simulink model "testing_C_functions_doubles_substituting_every_function"  (R2020b)
settings: Solver=FixedStepAuto  StartTime=0.0  StopTime=10  FixedStep=Ts  RelTol=1e-3
undefined symbols (not defined in the file or in its folder): A_frq_step, A_phase_step, DiscIntNeverNeededParam, f_rad, k_phi, ki, kp, N, t_frq_step, t_phase_step, Ts, V_g, var_noise
libraries: bach_library x24, simulink x16, dspsrcs4 x1
(part 1 of 2)
settings Model: Creator=Kasper Laustsen  LastModifiedBy=Kasper Laustsen
settings SFSimCC: SimCustomHeaderCode=|
  | #include "PLL_doubled.h"
  | #include "MAF_doubled.h"
settings SFSimCC: SimUserSources=|
  | PLL_doubled.c
  | MAF_doubled.c

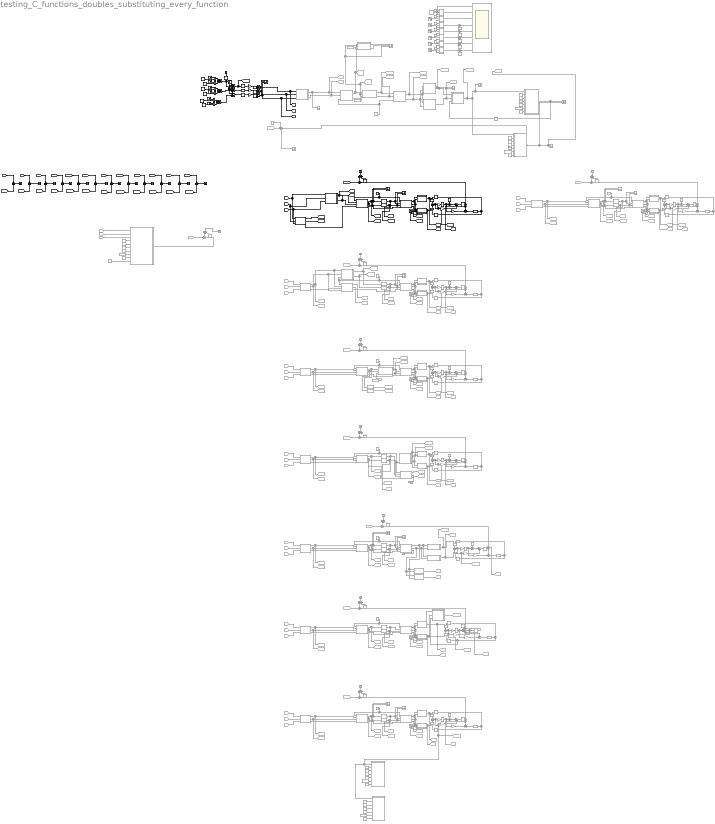
== system testing_C_functions_doubles_substituting_every_function ==
  note: Testing abc_to_alpha_beta
  note: TESTING abc_to_alphabeta
  note: MAF seems to be the limiting factor in terms of the code.
      | Experiment with changing the code inside of it to enable full simulation
  note: Noise
  note: Phase-jump
  note: Input signal incl. noise and phase- and frequency jump
  note: Frequency-jump
  note: MAF seems to be the limiting factor in terms of the code.
      | Experiment with changing the code inside of it to enable full simulation
  note: theta_pll
  note: theta_grid
  note: theta_pll
  note: theta_grid
  note: TESTING alphabeta_to_dq
  note: theta_pll
  note: theta_grid
  note: theta_grid
  note: theta_pll
  note: TESTING MAF
  note: theta_grid
  note: theta_pll
  note: TESTING dq_to_alphabeta
  note: theta_grid
  note: theta_pll
  note: TESTING cos_grid and sin_grid
  note: theta_grid
  note: theta_pll
  note: TESTING phase_detector
  note: theta_grid
  note: theta_pll
  note: TESTING pi_controller
  note: theta_grid
  note: theta_pll
  note: TRUE SIMULATION MODEL WITH DELAY
  Add{,1..5,7..10} (10 alike) : Sum
  Add{6,11..17} (8 alike) : Sum  Commented=on
  Chirp4 : dspsrcs4/Chirp  Commented=on  sweep=Linear  mode=Bidirectional  f0=0  f1=100  t1=2  Tsweep=2  phase=0  Ts=Ts  spf=1  datatype=Single  OutputFrames=off
  Constant{1..2,24,26,34,36,38,40,42,44,46,48} (12 alike) : Constant  Commented=on  Value=f_rad
  Constant{6,10,25,47,52} (5 alike) : Constant  Commented=on  Value=Ts
  Constant11 : Constant  Commented=on  Value=pi/2
  Constant12 : Constant  Commented=on  Value=6
  Constant13 : Constant  Commented=on  Value=10
  Constant14 : Constant  Commented=on  Value=8
  Constant{15..18,21..23} (7 alike) : Constant  Commented=on  Value=200
  Constant19 : Constant  Commented=on  Value=2
  Constant20 : Constant  Commented=on  Value=4
  Constant27 : Constant  Value=f_rad
  Constant28 : Constant  Value=-pi/2
  Constant{3,7,29,49,53} (5 alike) : Constant  Commented=on  Value=ki
  Constant{4,8,30,50,54} (5 alike) : Constant  Commented=on  Value=kp
  Constant{5,9,31,51,55} (5 alike) : Constant  Commented=on  Value=k_phi
  Constant{32..33,35,37,39,41,43,45} (8 alike) : Constant  Commented=on  Value=-pi/2
  Cos1 : Trigonometry  Operator=cos
  Cos{2..8} (7 alike) : Trigonometry  Commented=on  Operator=cos
  Delay : Delay  Commented=on  DelayLength=1  SampleTime=Ts
  Delay{1,3..8} (7 alike) : Delay  Commented=on  DelayLength=1
  Delay2 : Delay  DelayLength=1
  Derivative : Derivative
  Digital Clock{1..15} (15 alike) : DigitalClock  Commented=on  SampleTime=Ts
  Discrete FIR Filter{1,3,5..16} (14 alike) : DiscreteFir  Commented=on  Coefficients=[ones(1,round(N)).*1/N]  SampleTime=Ts
  Discrete FIR Filter2 : DiscreteFir  Coefficients=[ones(1,round(N)).*1/N]  SampleTime=Ts
  Discrete FIR Filter4 : DiscreteFir  Coefficients=[ones(1,round(N)).*1/N]  SampleTime=Ts
  Discrete-Time Integrator{1..2,5..16} (14 alike) : DiscreteIntegrator  Commented=on  IntegratorMethod=Integration: Trapezoidal  SampleTime=-1  ICPrevOutput=DiscIntNeverNeededParam  ICPrevScaledInput=DiscIntNeverNeededParam
  Discrete-Time Integrator3 : DiscreteIntegrator  IntegratorMethod=Integration: Trapezoidal  SampleTime=-1  ICPrevOutput=DiscIntNeverNeededParam  ICPrevScaledInput=DiscIntNeverNeededParam
  Discrete-Time Integrator4 : DiscreteIntegrator  IntegratorMethod=Integration: Trapezoidal  SampleTime=-1  ICPrevOutput=DiscIntNeverNeededParam  ICPrevScaledInput=DiscIntNeverNeededParam
  From{6,10,37,41,45,49,53,57} (8 alike) : From  Commented=on  GotoTag=B
  From{7,11,38,42,46,50,54,58} (8 alike) : From  Commented=on  GotoTag=C
  From{3,8,36,39,43,47,51,55,59} (9 alike) : From  Commented=on  GotoTag=phA_angle
  From{5,9,40,44,48,52,56,60} (8 alike) : From  Commented=on
  Gain{10..11,14,17,20,23,26} (7 alike) : Gain  Commented=on  Gain=k_phi
  Gain{2,12,15,18,21,24,27} (7 alike) : Gain  Commented=on  Gain=kp
  Gain{6,13,16,19,22,25,28} (7 alike) : Gain  Commented=on  Gain=ki
  Gain3 : Gain  Gain=V_g
  Gain4 : Gain  Gain=V_g
  Gain5 : Gain  Gain=V_g
  Gain7 : Gain  Gain=kp
  Gain8 : Gain  Gain=ki
  Gain9 : Gain  Gain=k_phi
  Goto{10,55,68,81,94,114} (6 alike) : Goto  Commented=on  GotoTag=d_pre_MAF
  Goto{40,48,61,87,100,107} (6 alike) : Goto  Commented=on  GotoTag=beta2
  Goto{41,49,62,75,88,101,108} (7 alike) : Goto  Commented=on  GotoTag=cosGrid
  Goto{5,50,63,76,89,102,109} (7 alike) : Goto  Commented=on  GotoTag=alpha1
  Goto{6,51,64,77,90,103,110} (7 alike) : Goto  Commented=on  GotoTag=sinGrid
  Goto{7,52,65,78,91,104,111} (7 alike) : Goto  Commented=on  GotoTag=anglePll
  Goto{8,53,66,79,92,105,112} (7 alike) : Goto  Commented=on  GotoTag=phaseError
  Goto{9,54,67,80,93,106,113} (7 alike) : Goto  Commented=on  GotoTag=beta1
  Goto{11,56,69,82,95,115} (6 alike) : Goto  Commented=on  GotoTag=q_pre_MAF
  Goto{12,44,57,70,83,96,116} (7 alike) : Goto  Commented=on  GotoTag=d_post_MAF
  Goto{38,45,58,71,84,97,117} (7 alike) : Goto  Commented=on  GotoTag=q_post_MAF
  Goto{39,46,59,85,98,118} (6 alike) : Goto  Commented=on  GotoTag=alpha2
  Goto13 : Goto  Commented=on  GotoTag=alpha1_C
  Goto14 : Goto  Commented=on  GotoTag=sinGrid_C
  Goto15 : Goto  Commented=on  GotoTag=anglePll_C
  Goto16 : Goto  Commented=on  GotoTag=phaseError_C
  Goto17 : Goto  Commented=on  GotoTag=beta1_C
  Goto18 : Goto  Commented=on  GotoTag=d_pre_MAF_C
  Goto19 : Goto  Commented=on  GotoTag=q_pre_MAF_C
  Goto20 : Goto  Commented=on  GotoTag=d_post_MAF_C
  Goto21 : Goto  Commented=on  GotoTag=q_post_MAF_C
  Goto22 : Goto  Commented=on  GotoTag=alpha2_C
  Goto23 : Goto  Commented=on  GotoTag=beta2_C
  Goto24 : Goto  Commented=on  GotoTag=cosGrid_C
  Goto42 : Goto  Commented=on  GotoTag=d_post_MAF_C
  Goto43 : Goto  Commented=on  GotoTag=q_post_MAF_C
  Goto47 : Goto  Commented=on  GotoTag=d_pre_MAF_C
  Goto60 : Goto  Commented=on  GotoTag=q_pre_MAF_C
  Goto72 : Goto  Commented=on  GotoTag=sinGrid_C
  Goto73 : Goto  Commented=on  GotoTag=alpha2_C
  Goto74 : Goto  Commented=on  GotoTag=cosGrid_C
  Goto86 : Goto  Commented=on  GotoTag=beta2_C
  Goto99 : Goto  Commented=on  GotoTag=phaseError_C
  MATLAB Function1 : MATLAB Function  Commented=on  TreatAsAtomicUnit=on
  MATLAB Function10 : MATLAB Function  Commented=on  TreatAsAtomicUnit=on
  MATLAB Function11 : MATLAB Function  Commented=on  TreatAsAtomicUnit=on
  MATLAB Function12 : MATLAB Function  Commented=on  TreatAsAtomicUnit=on
  MATLAB Function13 : MATLAB Function  Commented=on  TreatAsAtomicUnit=on
  MATLAB Function14 : MATLAB Function  Commented=on  TreatAsAtomicUnit=on
  MATLAB Function15 : MATLAB Function  Commented=on  TreatAsAtomicUnit=on
  MATLAB Function16 : MATLAB Function  Commented=on  TreatAsAtomicUnit=on
  MATLAB Function17 : MATLAB Function  Commented=on  TreatAsAtomicUnit=on
  MATLAB Function18 : MATLAB Function  Commented=on  TreatAsAtomicUnit=on
  MATLAB Function19 : MATLAB Function  TreatAsAtomicUnit=on
  MATLAB Function2 : MATLAB Function  Commented=on  TreatAsAtomicUnit=on
  MATLAB Function20 : MATLAB Function  TreatAsAtomicUnit=on
  MATLAB Function21 : MATLAB Function  Commented=on  TreatAsAtomicUnit=on
  MATLAB Function22 : MATLAB Function  Commented=on  TreatAsAtomicUnit=on
  MATLAB Function23 : MATLAB Function  Commented=on  TreatAsAtomicUnit=on
  MATLAB Function24 : MATLAB Function  Commented=on  TreatAsAtomicUnit=on
  MATLAB Function25 : MATLAB Function  Commented=on  TreatAsAtomicUnit=on
  MATLAB Function26 : MATLAB Function  Commented=on  TreatAsAtomicUnit=on
  MATLAB Function27 : MATLAB Function  Commented=on  TreatAsAtomicUnit=on
  MATLAB Function28 : MATLAB Function  Commented=on  TreatAsAtomicUnit=on
  MATLAB Function29 : MATLAB Function  Commented=on  TreatAsAtomicUnit=on
  MATLAB Function3 : MATLAB Function  Commented=on  TreatAsAtomicUnit=on
  MATLAB Function30 : MATLAB Function  Commented=on  TreatAsAtomicUnit=on
  MATLAB Function31 : MATLAB Function  Commented=on  TreatAsAtomicUnit=on
  MATLAB Function32 : MATLAB Function  Commented=on  TreatAsAtomicUnit=on
  MATLAB Function33 : MATLAB Function  Commented=on  TreatAsAtomicUnit=on
  MATLAB Function34 : MATLAB Function  Commented=on  TreatAsAtomicUnit=on
  MATLAB Function35 : MATLAB Function  Commented=on  TreatAsAtomicUnit=on
  MATLAB Function36 : MATLAB Function  Commented=on  TreatAsAtomicUnit=on
  MATLAB Function37 : MATLAB Function  Commented=on  TreatAsAtomicUnit=on
  MATLAB Function38 : MATLAB Function  Commented=on  TreatAsAtomicUnit=on
  MATLAB Function39 : MATLAB Function  Commented=on  TreatAsAtomicUnit=on
  MATLAB Function4 : MATLAB Function  Commented=on  TreatAsAtomicUnit=on
  MATLAB Function40 : MATLAB Function  Commented=on  TreatAsAtomicUnit=on
  MATLAB Function41 : MATLAB Function  Commented=on  TreatAsAtomicUnit=on
  MATLAB Function42 : MATLAB Function  Commented=on  TreatAsAtomicUnit=on
  MATLAB Function43 : MATLAB Function  Commented=on  TreatAsAtomicUnit=on
  MATLAB Function5 : MATLAB Function  Commented=on  TreatAsAtomicUnit=on
  MATLAB Function6 : MATLAB Function  Commented=on  TreatAsAtomicUnit=on
  MATLAB Function7 : MATLAB Function  Commented=on  TreatAsAtomicUnit=on
  MATLAB Function8 : MATLAB Function  Commented=on  TreatAsAtomicUnit=on
  MATLAB Function9 : MATLAB Function  TreatAsAtomicUnit=on
  Matrix Multiply{1,10..22} (14 alike) : Product  Commented=on
  Matrix Multiply{2..9} (8 alike) : Product
  Random Number : RandomNumber  Variance=var_noise  SampleTime=Ts
  Random Number1 : RandomNumber  Variance=var_noise  Seed=1  SampleTime=Ts
  Random Number2 : RandomNumber  Variance=var_noise  Seed=2  SampleTime=Ts
  Scope : Scope  Commented=on  NumInputPorts=3
  Scope1 : Scope  Commented=on
  Scope2 : Scope  Commented=on  NumInputPorts=8
  Scope3 : Scope  Commented=on
  Scope4 : Scope  Commented=on
  Scope5 : Scope  Commented=on  NumInputPorts=2
  Scope6 : Scope  Commented=on  NumInputPorts=2
  Scope8 : Scope  Commented=on  NumInputPorts=2
  Sin{1,3..5} (4 alike) : Trigonometry
  Sin{2,6..11} (7 alike) : Trigonometry  Commented=on
  Sine Wave14 : Sin  Commented=on  Frequency=f_rad*2.6  Phase=pi/2  SampleTime=Ts
  Sine Wave15 : Sin  Commented=on  Frequency=f_rad*2.8  Phase=pi/2  SampleTime=Ts
  Sine Wave16 : Sin  Commented=on  Frequency=f_rad*3  Phase=pi/2  SampleTime=Ts
  Sine Wave22 : Sin  Commented=on  Frequency=f_rad*2  Phase=pi/2  SampleTime=Ts
  Sine Wave23 : Sin  Commented=on  Frequency=f_rad*2.2  Phase=pi/2  SampleTime=Ts
  Sine Wave24 : Sin  Commented=on  Frequency=f_rad*2.4  Phase=pi/2  SampleTime=Ts
  Step : Step  Time=t_frq_step  Before=1  After=0  SampleTime=0
  Step1 : Step  Time=t_frq_step  SampleTime=0
  Step2 : Step  Time=t_frq_step  Before=1  After=0  SampleTime=0
  Step3 : Step  Time=t_frq_step  SampleTime=0
  Step4 : Step  Time=t_frq_step  Before=1  After=0  SampleTime=0
  Step5 : Step  Time=t_frq_step  SampleTime=0
  Sum : Sum  Commented=on  Inputs=+-|-
  Sum{1..4,9,15,33,38,43,48,53,58} (12 alike) : Sum  Commented=on  Inputs=|++
  Sum{10..14,16..22,25} (13 alike) : Sum  Inputs=+|-
  Sum23 : Sum  Inputs=-|+
  Sum24 : Sum  Inputs=++|
  Sum26 : Sum  Inputs=|++
  Sum27 : Sum  Inputs=+-|
  Sum{28..29,34,39,44,49,54} (7 alike) : Sum  Commented=on  Inputs=+-|
  Sum{6,30,35,40,45,50,55} (7 alike) : Sum  Commented=on  Inputs=-|+
  Sum{7,31,36,41,46,51,56} (7 alike) : Sum  Commented=on  Inputs=++|
  Sum{5,8,32,37,42,47,52,57} (8 alike) : Sum  Commented=on  Inputs=+|-
  Terminator{,2..15} (15 alike) : Terminator
  Terminator{1,16..29} (15 alike) : Terminator  Commented=on
  a_frq : simulink/Sources/Ramp  slope=f_rad  start=0  InitialOutput=0
  a_frq_step : simulink/Sources/Ramp  slope=f_rad*A_frq_step  start=t_frq_step  InitialOutput=t_frq_step*f_rad
  abc_to_alphabeta1 : bach_library/abc_to_alphabeta  SystemSampleTime=-1  VariantActivationTime=update diagram  Latency=0  AutoFrameSizeCalculation=off
  abc_to_alphabeta{2..8} (7 alike) : bach_library/abc_to_alphabeta  Commented=on  SystemSampleTime=-1  VariantActivationTime=update diagram  Latency=0  AutoFrameSizeCalculation=off
  alphabeta_to_dq1 : bach_library/alphabeta_to_dq  SystemSampleTime=-1  VariantActivationTime=update diagram  Latency=0  AutoFrameSizeCalculation=off
  alphabeta_to_dq{2..8} (7 alike) : bach_library/alphabeta_to_dq  Commented=on  SystemSampleTime=-1  VariantActivationTime=update diagram  Latency=0  AutoFrameSizeCalculation=off
  b_frq : simulink/Sources/Ramp  slope=f_rad  start=0  InitialOutput=-pi*2/3
  b_frq_step : simulink/Sources/Ramp  slope=f_rad*A_frq_step  start=t_frq_step  InitialOutput=t_frq_step*f_rad-pi*2/3
  c_frq : simulink/Sources/Ramp  slope=f_rad  start=0  InitialOutput=pi*2/3
  c_frq_step : simulink/Sources/Ramp  slope=f_rad*A_frq_step  start=t_frq_step  InitialOutput=t_frq_step*f_rad+pi*2/3
  dq_to_alphabeta1 : bach_library/dq_to_alphabeta  SystemSampleTime=-1  VariantActivationTime=update diagram  Latency=0  AutoFrameSizeCalculation=off
  dq_to_alphabeta{2..8} (7 alike) : bach_library/dq_to_alphabeta  Commented=on  SystemSampleTime=-1  VariantActivationTime=update diagram  Latency=0  AutoFrameSizeCalculation=off
  nominal frq{,1,3..9} (9 alike) : simulink/Sources/Ramp  Commented=on  slope=f_rad  start=0  InitialOutput=0
  nominal frq2 : simulink/Sources/Ramp  slope=f_rad  start=0  InitialOutput=0
  phase-jump : Step  Time=t_phase_step  After=A_phase_step  SampleTime=0
  phases : Scope  NumInputPorts=3
  post MAF1 : Scope  NumInputPorts=2
  post MAF{2,5,7..8} (4 alike) : Scope  Commented=on  NumInputPorts=2
  pre MAF1 : Scope  NumInputPorts=3
  pre MAF5 : Scope  Commented=on  NumInputPorts=3
  pre MAF7 : Scope  Commented=on  NumInputPorts=3
  pre MAF8 : Scope  Commented=on  NumInputPorts=3
  wires:
  MATLAB Function2/1(alpha) -> Goto13/1, MATLAB Function3/1(alpha), Scope4/1  "alpha1_C"
  Matrix Multiply4/1 -> Add5/2
  Matrix Multiply6/1 -> Add3/1
  Step2/1 -> Matrix Multiply2/1
  Matrix Multiply7/1 -> Add5/1
  Step4/1 -> Matrix Multiply4/1
  a_frq_step/1 -> Matrix Multiply6/2
  a_frq/1 -> Matrix Multiply5/2
  Step/1 -> Matrix Multiply5/1
  Sin5/1 -> Gain5/1  "theta_g"
  Gain5/1 -> Add9/1  "pc"
  Step5/1 -> Matrix Multiply7/1
  Matrix Multiply2/1 -> Add4/2
  Add5/1 -> Add2/2  "c_phase"
  c_frq_step/1 -> Matrix Multiply7/2
  b_frq/1 -> Matrix Multiply2/2
  Gain4/1 -> Add8/1  "pb"
  phase-jump/1 -> Add/1, Add2/1, Add1/1
  Add4/1 -> Add1/2  "b_phase"
  Add3/1 -> Add/2, Derivative/1  "a_phase"
  Random Number2/1 -> Add9/2
  b_frq_step/1 -> Matrix Multiply3/2
  Gain3/1 -> Add7/1  "pa"
  Sin4/1 -> Gain4/1  "theta_g"
  Add1/1 -> Sin4/1
  Random Number/1 -> Add7/2
  c_frq/1 -> Matrix Multiply4/2
  Add2/1 -> Sin5/1
  Random Number1/1 -> Add8/2
  Sin3/1 -> Gain3/1  "theta_g"
  Matrix Multiply5/1 -> Add3/2
  Step3/1 -> Matrix Multiply3/1
  Matrix Multiply3/1 -> Add4/1
  Step1/1 -> Matrix Multiply6/1
  Derivative/1 -> Terminator3/1  "omega_g"
  MATLAB Function4/2(beta) -> Goto23/1, MATLAB Function5/2(beta), MATLAB Function6/2(beta)  "beta2_C"
  MATLAB Function4/1(alpha) -> Goto22/1, MATLAB Function5/1(alpha), MATLAB Function6/1(alpha)  "alpha2_C"
  MATLAB Function5/1(cosGrid) -> Goto24/1, Scope8/1, MATLAB Function10/1(cosGrid)  "cosGrid_C"
  MATLAB Function6/1(sinGrid) -> MATLAB Function10/2(sinGrid), Scope8/2, Goto14/1  "sinGric_C"
  Constant2/1 -> MATLAB Function8/2(feedForward)
  Constant1/1 -> MATLAB Function7/2(feedForward)
  Digital Clock1/1 -> MATLAB Function7/6(t)
  Constant9/1 -> MATLAB Function8/5(kPhi)
  Digital Clock2/1 -> MATLAB Function8/6(t)
  Constant8/1 -> MATLAB Function8/4(kp)
  Constant6/1 -> MATLAB Function7/7(Ts)
  Constant7/1 -> MATLAB Function8/3(ki)
  Constant5/1 -> MATLAB Function7/5(kPhi)
  Constant10/1 -> MATLAB Function8/7(Ts)
  Constant4/1 -> MATLAB Function7/4(kp)
  Constant3/1 -> MATLAB Function7/3(ki)
  MATLAB Function7/1(anglePll) -> Sum/3, Scope6/2, Goto15/1, Scope5/1  "anglePll"
  nominal frq/1 -> MATLAB Function3/3(angle), MATLAB Function4/3(angle)
  MATLAB Function10/1(phaseError) -> Goto16/1, MATLAB Function7/1(phaseError), Scope3/1, MATLAB Function8/1(phaseError)  "phaseError_C"
  MATLAB Function8/1(anglePllComp) -> Delay/1, Scope6/1
  Constant11/1 -> Sum/2
  Sum/1 -> Scope1/1  "Angle_error_offset"
  MATLAB Function3/2(q) -> MATLAB Function18/2(sample2), Scope/3, MATLAB Function1/2(sample2), Goto19/1  "q_pre_MAF_C"
  Sum15/1 -> Scope2/8  "sin 150 Hz MAFed"
  Constant20/1 -> Sum2/2
  MATLAB Function12/1(y) -> Scope2/3  "sin 100 Hz MAFed"
  Constant19/1 -> Sum1/2
  MATLAB Function15/1(y) -> Sum3/1
  MATLAB Function14/1(y) -> Sum2/1
  Sine Wave14/1 -> MATLAB Function15/2(sample)
  Constant13/1 -> Sum15/2
  MATLAB Function17/1(y) -> Sum15/1
  MATLAB Function11/1(y) -> Scope2/2  "chirp MAFed"
  Sum2/1 -> Scope2/5  "sin 120 Hz MAFed"
  Sum3/1 -> Scope2/6  "sin 130 Hz MAFed"
  Chirp4/1 -> MATLAB Function11/2(sample), Scope2/1  "pa"
  Sine Wave22/1 -> MATLAB Function12/2(sample)
  Sine Wave15/1 -> MATLAB Function16/2(sample)
  MATLAB Function16/1(y) -> Sum4/1
  Sine Wave23/1 -> MATLAB Function13/2(sample)
  Constant14/1 -> Sum4/2
  Sum1/1 -> Scope2/4  "sin 110 Hz MAFed"
  MATLAB Function13/1(y) -> Sum1/1
  Sine Wave16/1 -> MATLAB Function17/2(sample)  "theta_g"
  Constant12/1 -> Sum3/2
  Sine Wave24/1 -> MATLAB Function14/2(sample)
  Sum4/1 -> Scope2/7  "sin 140 Hz MAFed"
  Constant15/1 -> MATLAB Function11/1(len)
  Digital Clock3/1 -> MATLAB Function11/3(t)
  Digital Clock4/1 -> MATLAB Function12/3(t)
  Constant16/1 -> MATLAB Function12/1(len)
  Digital Clock5/1 -> MATLAB Function13/3(t)
  Constant17/1 -> MATLAB Function13/1(len)
  Digital Clock6/1 -> MATLAB Function14/3(t)
  Constant18/1 -> MATLAB Function14/1(len)
  Digital Clock7/1 -> MATLAB Function15/3(t)
  Constant21/1 -> MATLAB Function15/1(len)
  Digital Clock8/1 -> MATLAB Function16/3(t)
  Constant22/1 -> MATLAB Function16/1(len)
  Digital Clock9/1 -> MATLAB Function17/3(t)
  Constant23/1 -> MATLAB Function17/1(len)
  MATLAB Function3/1(d) -> MATLAB Function18/1(sample1), Goto18/1, MATLAB Function1/1(sample1)  "d_pre_MAF_C"
  MATLAB Function18/1(y1) -> Goto20/1, MATLAB Function4/1(d)  "d_post_MAF_C"
  MATLAB Function18/2(y2) -> Goto21/1, MATLAB Function4/2(q)  "q_post_MAF_C"
  MATLAB Function2/2(beta) -> MATLAB Function3/2(beta), Goto17/1  "beta1_C"
  [alpha1] -> Sum10/1
  [alpha1_C] -> Sum10/2
  [beta1] -> Sum11/1
  [beta1_C] -> Sum11/2
  [d_pre_MAF] -> Sum12/1
  [d_pre_MAF_C] -> Sum12/2
  [q_pre_MAF_C] -> Sum13/2
  [q_pre_MAF] -> Sum13/1
  [d_post_MAF] -> Sum14/1
  [d_post_MAF_C] -> Sum14/2
  [q_post_MAF] -> Sum16/1
  [q_post_MAF_C] -> Sum16/2
  [alpha2] -> Sum17/1
  [alpha2_C] -> Sum17/2
  [beta2] -> Sum18/1
  [beta2_C] -> Sum18/2
  [cosGrid] -> Sum19/1
  [cosGrid_C] -> Sum19/2
  [sinGrid] -> Sum20/1
  [sinGrid_C] -> Sum20/2
  [phaseError] -> Sum21/1
  [phaseError_C] -> Sum21/2
  [anglePll] -> Sum22/1
  [anglePll_C] -> Sum22/2
  Sum10/1 -> Terminator/1  "diff_alpha1"
  Sum11/1 -> Terminator4/1  "diff_beta1"
  Sum12/1 -> Terminator5/1  "diff_d_pre_MAF"
  Sum13/1 -> Terminator6/1  "diff_q_pre_MAF"
  Sum14/1 -> Terminator7/1  "diff_d_post_MAF"
  Sum16/1 -> Terminator8/1  "diff_q_post_MAF"
  Sum17/1 -> Terminator9/1  "diff_alpha2"
  Sum18/1 -> Terminator10/1  "diff_beta2"
  Sum19/1 -> Terminator11/1  "diff_cosGrid"
  Sum20/1 -> Terminator12/1  "diff_sinGrid"
  Sum21/1 -> Terminator13/1  "diff_phaseError"
  Sum22/1 -> Terminator14/1  "diff_anglePll"
  Delay/1 -> MATLAB Function10/3(anglePllComp)
  Sum27/1 -> Delay2/1  "theta_comp"
  Sum25/1 -> Add10/1  "theta_err_sim"
  alphabeta_to_dq1/3 -> dq_to_alphabeta1/4
  Gain7/1 -> Sum26/2
  Gain8/1 -> Discrete-Time Integrator3/1
  Constant27/1 -> Sum24/1
  dq_to_alphabeta1/3 -> Terminator15/1
  Cos1/1 -> Matrix Multiply9/2  "cos_pll"
  MATLAB Function20/1(sin_grid) -> [sinGrid], Matrix Multiply9/1  "sin_grid"
  Gain9/1 -> Sum27/2  "k_phi"
  Add/1 -> [phA_angle], Sin3/1  "pha_angle"
  abc_to_alphabeta1/3 -> alphabeta_to_dq1/4
  abc_to_alphabeta1/1 -> [alpha1]  "alpha1_sim"
  Discrete FIR Filter4/1 -> [d_post_MAF], post MAF1/1, dq_to_alphabeta1/2  "d_post_MAF"
  abc_to_alphabeta1/2 -> [beta1]  "beta1_sim"
  dq_to_alphabeta1/2 -> [beta2], MATLAB Function20/1(beta), MATLAB Function19/2(beta)  "beta2"
  nominal frq2/1 -> dq_to_alphabeta1/1, alphabeta_to_dq1/1
  Add8/1 -> phases/2, [B], MATLAB Function2/2(b)  "pb"
  Sin1/1 -> Matrix Multiply8/2  "sin_pll"
  Discrete-Time Integrator4/1 -> Sum27/1, [anglePll], Sum25/2  "theta"
  Sum24/1 -> Sum26/1
  alphabeta_to_dq1/1 -> [d_pre_MAF], pre MAF1/1, Discrete FIR Filter4/1  "d_pre_MAF"
  Sum26/1 -> Discrete-Time Integrator4/1  "omega"
  Discrete FIR Filter2/1 -> [q_post_MAF], post MAF1/2, dq_to_alphabeta1/3  "q_post_MAF"
  Add10/1 -> Terminator2/1  "theta_err_sim_offset_delay"
  Matrix Multiply9/1 -> Sum23/2  "sin_grid_cos_pll"
  alphabeta_to_dq1/2 -> [q_pre_MAF], Discrete FIR Filter2/1, pre MAF1/2  "q_pre_MAF"
  dq_to_alphabeta1/1 -> MATLAB Function19/1(alpha), [alpha2], MATLAB Function20/2(alpha)  "alpha2"
  Add9/1 -> [C], MATLAB Function2/3(c), phases/3  "pc"
  Matrix Multiply8/1 -> Sum23/1  "cos_grid_sin_pll"
  Constant28/1 -> Add10/2
  Discrete-Time Integrator3/1 -> Sum24/2, Gain9/1
  Add7/1 -> [A], MATLAB Function2/1(a), phases/1  "pa"
  MATLAB Function19/1(cos_grid) -> [cosGrid], Matrix Multiply8/1  "cos_grid"
  Sum23/1 -> Gain8/1, [phaseError], Gain7/1  "phaseError"
  Delay2/1 -> Sin1/1, Cos1/1
  From3/1 -> Sum/1
  [phA_angle] -> Sum25/1
  [C] -> MATLAB Function9/3(c), abc_to_alphabeta1/3
  [B] -> MATLAB Function9/2(b), abc_to_alphabeta1/2
  [A] -> MATLAB Function9/1(a), abc_to_alphabeta1/1
  Digital Clock10/1 -> MATLAB Function1/3(t)
  MATLAB Function1/1(y1) -> Scope/1  "d_post_maf_C"
  MATLAB Function1/2(y2) -> Scope/2  "q_post_maf_C"
  Digital Clock11/1 -> MATLAB Function18/3(t)
  Constant25/1 -> MATLAB Function21/9(Ts)
  Constant30/1 -> MATLAB Function21/6(kp)
  Constant31/1 -> MATLAB Function21/7(kPhi)
  Constant29/1 -> MATLAB Function21/5(ki)
  Constant26/1 -> MATLAB Function21/4(feedForward)
  Digital Clock12/1 -> MATLAB Function21/8(t)
  From7/1 -> MATLAB Function21/3(c)
  From6/1 -> MATLAB Function21/2(b)
  From5/1 -> MATLAB Function21/1(a)
  nominal frq1/1 -> MATLAB Function21/10(angle)
  From8/1 -> Sum5/1
  Add6/1 -> Terminator1/1  "Angle Error C sammensat"
  Sum5/1 -> Add6/1  "theta_err_sim"
  MATLAB Function21/1(anglePll) -> Sum5/2  "theta"
  Constant32/1 -> Add6/2
  Add11/1 -> Terminator17/1  "theta_err_sim_offset_delay"
  From11/1 -> abc_to_alphabeta2/3
  From36/1 -> Sum8/1
  From9/1 -> abc_to_alphabeta2/1
  From10/1 -> abc_to_alphabeta2/2
  Sum6/1 -> Gain6/1, Goto8/1, Gain2/1  "phaseError"
  Delay1/1 -> Sin2/1, Cos2/1
  Matrix Multiply1/1 -> Sum6/1  "cos_grid_sin_pll"
  dq_to_alphabeta2/1 -> MATLAB Function22/1(alpha), Goto39/1, MATLAB Function23/2(alpha)  "alpha2"
  Matrix Multiply10/1 -> Sum6/2  "sin_grid_cos_pll"
  alphabeta_to_dq2/2 -> Goto11/1  "q_pre_MAF_sim"
  alphabeta_to_dq2/1 -> Goto10/1  "d_pre_MAF_sim"
  Constant33/1 -> Add11/2
  Discrete FIR Filter3/1 -> Goto12/1, post MAF2/1, dq_to_alphabeta2/2  "d_post_MAF"
  Discrete-Time Integrator2/1 -> Sum28/1, Goto7/1, Sum8/2  "theta"
  abc_to_alphabeta2/2 -> alphabeta_to_dq2/3, MATLAB Function34/2(beta), Goto9/1  "beta1"
  abc_to_alphabeta2/3 -> alphabeta_to_dq2/4
  Sin2/1 -> Matrix Multiply1/2  "sin_pll"
  MATLAB Function23/1(sin_grid) -> Goto6/1, Matrix Multiply10/1  "sin_grid"
  nominal frq3/1 -> dq_to_alphabeta2/1, alphabeta_to_dq2/1, MATLAB Function34/3(angle)
  Discrete-Time Integrator1/1 -> Sum7/2, Gain10/1
  Gain10/1 -> Sum28/2  "k_phi"
  Constant24/1 -> Sum7/1
  Gain6/1 -> Discrete-Time Integrator1/1
  alphabeta_to_dq2/3 -> dq_to_alphabeta2/4
  Gain2/1 -> Sum9/2
  dq_to_alphabeta2/3 -> Terminator16/1
  Sum8/1 -> Add11/1  "theta_err_sim"
  Sum28/1 -> Delay1/1  "theta_comp"
  MATLAB Function22/1(cos_grid) -> Goto41/1, Matrix Multiply1/1  "cos_grid"
  Cos2/1 -> Matrix Multiply10/2  "cos_pll"
  Sum7/1 -> Sum9/1
  dq_to_alphabeta2/2 -> Goto40/1, MATLAB Function23/1(beta), MATLAB Function22/2(beta)  "beta2"
  abc_to_alphabeta2/1 -> alphabeta_to_dq2/2, MATLAB Function34/1(alpha), Goto5/1  "alpha1"
  Sum9/1 -> Discrete-Time Integrator2/1  "omega"
  Discrete FIR Filter1/1 -> Goto38/1, post MAF2/2, dq_to_alphabeta2/3  "q_post_MAF"
  Sum32/1 -> Add12/1  "theta_err_sim"
  dq_to_alphabeta3/3 -> Terminator18/1
  Gain12/1 -> Sum33/2
  MATLAB Function24/1(cos_grid) -> Goto49/1, Matrix Multiply11/1  "cos_grid"
  Sum29/1 -> Delay3/1  "theta_comp"
  Gain11/1 -> Sum29/2  "k_phi"
  Constant34/1 -> Sum31/1
  Discrete-Time Integrator5/1 -> Sum31/2, Gain11/1
  nominal frq4/1 -> dq_to_alphabeta3/1, alphabeta_to_dq3/1
  Gain13/1 -> Discrete-Time Integrator5/1
  alphabeta_to_dq3/3 -> dq_to_alphabeta3/4
  MATLAB Function25/1(sin_grid) -> Goto51/1, Matrix Multiply12/1  "sin_grid"
  abc_to_alphabeta3/3 -> alphabeta_to_dq3/4
  Sin6/1 -> Matrix Multiply11/2  "sin_pll"
  Discrete FIR Filter6/1 -> Goto44/1  "d_post_MAF_sim"
  alphabeta_to_dq3/1 -> MATLAB Function37/1(sample1), Discrete FIR Filter6/1  "d_pre_MAF"
  abc_to_alphabeta3/2 -> alphabeta_to_dq3/3, Goto54/1  "beta1"
  Matrix Multiply12/1 -> Sum30/2  "sin_grid_cos_pll"
  Matrix Multiply11/1 -> Sum30/1  "cos_grid_sin_pll"
  Delay3/1 -> Sin6/1, Cos3/1
  Sum30/1 -> Gain13/1, Goto53/1, Gain12/1  "phaseError"
  alphabeta_to_dq3/2 -> Discrete FIR Filter5/1, MATLAB Function37/2(sample2)  "q_pre_MAF"
  From39/1 -> Sum32/1
  Constant35/1 -> Add12/2
  From40/1 -> abc_to_alphabeta3/1
  From37/1 -> abc_to_alphabeta3/2
  From38/1 -> abc_to_alphabeta3/3
  abc_to_alphabeta3/1 -> alphabeta_to_dq3/2, Goto50/1  "alpha1"
  Discrete-Time Integrator6/1 -> Sum29/1, Goto52/1, Sum32/2  "theta"
  dq_to_alphabeta3/2 -> Goto48/1, MATLAB Function25/1(beta), MATLAB Function24/2(beta)  "beta2"
  Discrete FIR Filter5/1 -> Goto45/1  "q_post_MAF_sim"
  Sum33/1 -> Discrete-Time Integrator6/1  "omega"
  Cos3/1 -> Matrix Multiply12/2  "cos_pll"
  Sum31/1 -> Sum33/1
  dq_to_alphabeta3/1 -> MATLAB Function24/1(alpha), Goto46/1, MATLAB Function25/2(alpha)  "alpha2"
  Add12/1 -> Terminator19/1  "theta_err_sim_offset_delay"
  Sum37/1 -> Add13/1  "theta_err_sim"
  dq_to_alphabeta4/3 -> Terminator20/1
  Gain15/1 -> Sum38/2
  MATLAB Function26/1(cos_grid) -> Goto62/1, Matrix Multiply13/1  "cos_grid"
  Sum34/1 -> Delay4/1  "theta_comp"
  Gain14/1 -> Sum34/2  "k_phi"
  Constant36/1 -> Sum36/1
  Discrete-Time Integrator7/1 -> Sum36/2, Gain14/1
  nominal frq5/1 -> dq_to_alphabeta4/1, MATLAB Function38/3(angle), alphabeta_to_dq4/1
  Gain16/1 -> Discrete-Time Integrator7/1
  alphabeta_to_dq4/3 -> dq_to_alphabeta4/4
  MATLAB Function27/1(sin_grid) -> Goto64/1, Matrix Multiply14/1  "sin_grid"
  abc_to_alphabeta4/3 -> alphabeta_to_dq4/4
  Sin7/1 -> Matrix Multiply13/2  "sin_pll"
  Discrete FIR Filter8/1 -> Goto57/1, dq_to_alphabeta4/2  "d_post_MAF"
  alphabeta_to_dq4/1 -> Goto55/1, Discrete FIR Filter8/1  "d_pre_MAF"
  abc_to_alphabeta4/2 -> alphabeta_to_dq4/3, Goto67/1  "beta1"
  Matrix Multiply14/1 -> Sum35/2  "sin_grid_cos_pll"
  Matrix Multiply13/1 -> Sum35/1  "cos_grid_sin_pll"
  Delay4/1 -> Sin7/1, Cos4/1
  Sum35/1 -> Gain16/1, Goto66/1, Gain15/1  "phaseError"
  alphabeta_to_dq4/2 -> Goto56/1, Discrete FIR Filter7/1  "q_pre_MAF"
  From43/1 -> Sum37/1
  Constant37/1 -> Add13/2
  From44/1 -> abc_to_alphabeta4/1
  From41/1 -> abc_to_alphabeta4/2
  From42/1 -> abc_to_alphabeta4/3
  abc_to_alphabeta4/1 -> alphabeta_to_dq4/2, Goto63/1  "alpha1"
  Discrete-Time Integrator8/1 -> Sum34/1, Goto65/1, Sum37/2  "theta"
  dq_to_alphabeta4/2 -> Goto61/1  "beta2_sim"
  Discrete FIR Filter7/1 -> Goto58/1, dq_to_alphabeta4/3  "q_post_MAF"
  Sum38/1 -> Discrete-Time Integrator8/1  "omega"
  Cos4/1 -> Matrix Multiply14/2  "cos_pll"
  Sum36/1 -> Sum38/1
  dq_to_alphabeta4/1 -> Goto59/1  "alpha2_sim"
  Add13/1 -> Terminator21/1  "theta_err_sim_offset_delay"
  Sum42/1 -> Add14/1  "theta_err_sim"
  dq_to_alphabeta5/3 -> Terminator22/1
  Gain18/1 -> Sum43/2
  MATLAB Function28/1(cos_grid) -> Goto75/1  "cos_grid_sim"
  Sum39/1 -> Delay5/1  "theta_comp"
  Gain17/1 -> Sum39/2  "k_phi"
  Constant38/1 -> Sum41/1
  Discrete-Time Integrator9/1 -> Sum41/2, Gain17/1
  nominal frq6/1 -> dq_to_alphabeta5/1, alphabeta_to_dq5/1
  Gain19/1 -> Discrete-Time Integrator9/1
  alphabeta_to_dq5/3 -> dq_to_alphabeta5/4
  MATLAB Function29/1(sin_grid) -> Goto77/1  "sin_grid_sim"
  abc_to_alphabeta5/3 -> alphabeta_to_dq5/4
  Sin8/1 -> Matrix Multiply15/2  "sin_pll"
  Discrete FIR Filter10/1 -> Goto70/1, post MAF5/1, dq_to_alphabeta5/2  "d_post_MAF"
  alphabeta_to_dq5/1 -> Goto68/1, pre MAF5/1, Discrete FIR Filter10/1  "d_pre_MAF"
  abc_to_alphabeta5/2 -> alphabeta_to_dq5/3, Goto80/1  "beta1"
  Matrix Multiply16/1 -> Sum40/2  "sin_grid_cos_pll"
  Matrix Multiply15/1 -> Sum40/1  "cos_grid_sin_pll"
  Delay5/1 -> Sin8/1, Cos5/1
  Sum40/1 -> Gain19/1, Gain18/1, Goto79/1  "phaseError"
  alphabeta_to_dq5/2 -> Goto69/1, Discrete FIR Filter9/1, pre MAF5/2  "q_pre_MAF"
  From47/1 -> Sum42/1
  Constant39/1 -> Add14/2
  From48/1 -> abc_to_alphabeta5/1
  From45/1 -> abc_to_alphabeta5/2
  From46/1 -> abc_to_alphabeta5/3
  abc_to_alphabeta5/1 -> alphabeta_to_dq5/2, Goto76/1  "alpha1"
  Discrete-Time Integrator10/1 -> Sum42/2, Goto78/1, Sum39/1  "theta"
  dq_to_alphabeta5/2 -> MATLAB Function40/2(beta), MATLAB Function39/2(beta), MATLAB Function29/1(beta), MATLAB Function28/2(beta)  "beta2"
  Discrete FIR Filter9/1 -> Goto71/1, post MAF5/2, dq_to_alphabeta5/3  "q_post_MAF"
  Sum43/1 -> Discrete-Time Integrator10/1  "omega"
  Cos5/1 -> Matrix Multiply16/2  "cos_pll"
  Sum41/1 -> Sum43/1
  dq_to_alphabeta5/1 -> MATLAB Function40/1(alpha), MATLAB Function39/1(alpha), MATLAB Function28/1(alpha), MATLAB Function29/2(alpha)  "alpha2"
  Add14/1 -> Terminator23/1  "theta_err_sim_offset_delay"
  Sum47/1 -> Add15/1  "theta_err_sim"
  dq_to_alphabeta6/3 -> Terminator24/1
  Gain21/1 -> Sum48/2
  MATLAB Function30/1(cos_grid) -> Matrix Multiply17/1, Goto88/1, MATLAB Function41/1(cosGrid)  "cos_grid"
  Sum44/1 -> Delay6/1  "theta_comp"
  Gain20/1 -> Sum44/2  "k_phi"
  Constant40/1 -> Sum46/1
  Discrete-Time Integrator11/1 -> Sum46/2, Gain20/1
  nominal frq7/1 -> dq_to_alphabeta6/1, alphabeta_to_dq6/1
  Gain22/1 -> Discrete-Time Integrator11/1
  alphabeta_to_dq6/3 -> dq_to_alphabeta6/4
  MATLAB Function31/1(sin_grid) -> Goto90/1, MATLAB Function41/2(sinGrid), Matrix Multiply18/1  "sin_grid"
  abc_to_alphabeta6/3 -> alphabeta_to_dq6/4
  Sin9/1 -> Matrix Multiply17/2  "sin_pll"
  Discrete FIR Filter12/1 -> Goto83/1, dq_to_alphabeta6/2  "d_post_MAF"
  alphabeta_to_dq6/1 -> Goto81/1, Discrete FIR Filter12/1  "d_pre_MAF"
  abc_to_alphabeta6/2 -> alphabeta_to_dq6/3, Goto93/1  "beta1"
  Matrix Multiply18/1 -> Sum45/2  "sin_grid_cos_pll"
  Matrix Multiply17/1 -> Sum45/1  "cos_grid_sin_pll"
  Sum45/1 -> Gain22/1, Gain21/1, Goto92/1  "phaseError_sim"
  alphabeta_to_dq6/2 -> Goto82/1, Discrete FIR Filter11/1  "q_pre_MAF"
  From51/1 -> Sum47/1
  Constant41/1 -> Add15/2
  From52/1 -> abc_to_alphabeta6/1
  From49/1 -> abc_to_alphabeta6/2
  From50/1 -> abc_to_alphabeta6/3
  abc_to_alphabeta6/1 -> alphabeta_to_dq6/2, Goto89/1  "alpha1"
  Discrete-Time Integrator12/1 -> Sum44/1, Goto91/1, Sum47/2  "theta"
  dq_to_alphabeta6/2 -> Goto87/1, MATLAB Function31/1(beta), MATLAB Function30/2(beta)  "beta2"
  Discrete FIR Filter11/1 -> Goto84/1, dq_to_alphabeta6/3  "q_post_MAF"
  Sum48/1 -> Discrete-Time Integrator12/1  "omega"
  Cos6/1 -> Matrix Multiply18/2  "cos_pll"
  Sum46/1 -> Sum48/1
  dq_to_alphabeta6/1 -> MATLAB Function30/1(alpha), Goto85/1, MATLAB Function31/2(alpha)  "alpha2"
  Add15/1 -> Terminator25/1  "theta_err_sim_offset_delay"
  Sum52/1 -> Add16/1  "theta_err_sim"
  dq_to_alphabeta7/3 -> Terminator26/1
  Gain24/1 -> Sum53/2
  MATLAB Function32/1(cos_grid) -> Goto101/1, Matrix Multiply19/1  "cos_grid"
  Sum49/1 -> Delay7/1  "theta_comp"
  Gain23/1 -> Sum49/2  "k_phi"
  Constant42/1 -> Sum51/1
  Discrete-Time Integrator13/1 -> Sum51/2, Gain23/1
  nominal frq8/1 -> dq_to_alphabeta7/1, alphabeta_to_dq7/1
  Gain25/1 -> Discrete-Time Integrator13/1
  alphabeta_to_dq7/3 -> dq_to_alphabeta7/4
  MATLAB Function33/1(sin_grid) -> Goto103/1, Matrix Multiply20/1  "sin_grid"
  abc_to_alphabeta7/3 -> alphabeta_to_dq7/4
  Sin10/1 -> Matrix Multiply19/2  "sin_pll"
  Discrete FIR Filter14/1 -> Goto96/1, post MAF7/1, dq_to_alphabeta7/2  "d_post_MAF"
  alphabeta_to_dq7/1 -> Goto94/1, pre MAF7/1, Discrete FIR Filter14/1  "d_pre_MAF"
  abc_to_alphabeta7/2 -> alphabeta_to_dq7/3, Goto106/1  "beta1"
  Matrix Multiply20/1 -> Sum50/2  "sin_grid_cos_pll"
  Matrix Multiply19/1 -> Sum50/1  "cos_grid_sin_pll"
  Delay7/1 -> Sin10/1, Cos7/1
  alphabeta_to_dq7/2 -> Goto95/1, Discrete FIR Filter13/1, pre MAF7/2  "q_pre_MAF"
  From55/1 -> Sum52/1
  Constant43/1 -> Add16/2
  From56/1 -> abc_to_alphabeta7/1
  From53/1 -> abc_to_alphabeta7/2
  From54/1 -> abc_to_alphabeta7/3
  abc_to_alphabeta7/1 -> alphabeta_to_dq7/2, Goto102/1  "alpha1"
  Discrete-Time Integrator14/1 -> Sum49/1, Goto104/1, Sum52/2  "theta"
  dq_to_alphabeta7/2 -> Goto100/1, MATLAB Function33/1(beta), MATLAB Function32/2(beta)  "beta2"
  Discrete FIR Filter13/1 -> Goto97/1, post MAF7/2, dq_to_alphabeta7/3  "q_post_MAF"
  Sum53/1 -> Discrete-Time Integrator14/1  "omega"
  Cos7/1 -> Matrix Multiply20/2  "cos_pll"
  Sum51/1 -> Sum53/1
  dq_to_alphabeta7/1 -> MATLAB Function32/1(alpha), Goto98/1, MATLAB Function33/2(alpha)  "alpha2"
  Add16/1 -> Terminator27/1  "theta_err_sim_offset_delay"
  dq_to_alphabeta8/1 -> MATLAB Function35/1(alpha), Goto118/1, MATLAB Function36/2(alpha)  "alpha2_sim"
  Add17/1 -> Terminator29/1  "theta_err_sim_offset_delay"
  Sum58/1 -> Discrete-Time Integrator16/1  "omega"
  Cos8/1 -> Matrix Multiply22/2  "cos_pll"
  Discrete FIR Filter15/1 -> Goto117/1, post MAF8/2, dq_to_alphabeta8/3  "q_post_MAF_sim"
  Sum56/1 -> Sum58/1
  dq_to_alphabeta8/2 -> Goto107/1, MATLAB Function36/1(beta), MATLAB Function35/2(beta)  "beta2_sim"
  Discrete-Time Integrator16/1 -> Sum54/1, Goto111/1, Sum57/2  "theta"
  Constant45/1 -> Add17/2
  From60/1 -> abc_to_alphabeta8/1
  From59/1 -> Sum57/1
  alphabeta_to_dq8/2 -> Goto115/1, Discrete FIR Filter15/1, pre MAF8/2  "q_pre_MAF_sim"
  abc_to_alphabeta8/1 -> alphabeta_to_dq8/2, Goto109/1  "alpha1_sim"
  Delay8/1 -> Sin11/1, Cos8/1
  From58/1 -> abc_to_alphabeta8/3
  alphabeta_to_dq8/1 -> Goto114/1, pre MAF8/1, Discrete FIR Filter16/1  "d_pre_MAF_sim"
  Sum55/1 -> Gain28/1, Goto112/1, Gain27/1  "phaseError_sim"
  Matrix Multiply22/1 -> Sum55/2  "sin_grid_cos_pll"
  abc_to_alphabeta8/2 -> alphabeta_to_dq8/3, Goto113/1  "beta1_sim"
  abc_to_alphabeta8/3 -> alphabeta_to_dq8/4
  Sin11/1 -> Matrix Multiply21/2  "sin_pll"
  Discrete FIR Filter16/1 -> Goto116/1, post MAF8/1, dq_to_alphabeta8/2  "d_post_MAF_sim"
  MATLAB Function36/1(sin_grid) -> Goto110/1, Matrix Multiply22/1  "sin_grid_sim"
  Matrix Multiply21/1 -> Sum55/1  "cos_grid_sin_pll"
  nominal frq9/1 -> dq_to_alphabeta8/1, alphabeta_to_dq8/1
  Discrete-Time Integrator15/1 -> Sum56/2, Gain26/1
  alphabeta_to_dq8/3 -> dq_to_alphabeta8/4
  Gain28/1 -> Discrete-Time Integrator15/1
  Constant44/1 -> Sum56/1
  Sum57/1 -> Add17/1  "theta_err_sim"
  Gain26/1 -> Sum54/2  "k_phi"
  Sum54/1 -> Delay8/1  "theta_comp"
  From57/1 -> abc_to_alphabeta8/2
  dq_to_alphabeta8/3 -> Terminator28/1
  MATLAB Function35/1(cos_grid) -> Goto108/1, Matrix Multiply21/1  "cos_grid_sim"
  Gain27/1 -> Sum58/2
  Constant52/1 -> MATLAB Function42/7(Ts)
  Constant47/1 -> MATLAB Function43/7(Ts)
  Constant51/1 -> MATLAB Function42/5(kPhi)
  Constant48/1 -> MATLAB Function43/2(feedForward)
  Constant54/1 -> MATLAB Function43/4(kp)
  Constant55/1 -> MATLAB Function43/5(kPhi)
  Constant46/1 -> MATLAB Function42/2(feedForward)
  Constant53/1 -> MATLAB Function43/3(ki)
  Constant50/1 -> MATLAB Function42/4(kp)
  Digital Clock15/1 -> MATLAB Function43/6(t)
  Sum50/1 -> Gain25/1, Gain24/1, Goto105/1, MATLAB Function43/1(phaseError), MATLAB Function42/1(phaseError)  "phaseError_C"
  Digital Clock14/1 -> MATLAB Function42/6(t)
  Constant49/1 -> MATLAB Function42/3(ki)
  MATLAB Function9/2(beta) -> [beta1_C], alphabeta_to_dq1/3  "beta1_C"
  MATLAB Function9/1(alpha) -> [alpha1_C], alphabeta_to_dq1/2  "alpha1_C"
  MATLAB Function34/1(d) -> Discrete FIR Filter3/1, Goto47/1  "d_pre_MAF_C"
  MATLAB Function34/2(q) -> Goto60/1, Discrete FIR Filter1/1  "q_pre_MAF_C"
  Digital Clock13/1 -> MATLAB Function37/3(t)
  MATLAB Function37/1(y1) -> Goto42/1, dq_to_alphabeta3/2  "d_post_MAF_C"
  MATLAB Function37/2(y2) -> dq_to_alphabeta3/3, Goto43/1  "q_post_MAF_C"
  MATLAB Function38/2(beta) -> Goto86/1, MATLAB Function26/2(beta), MATLAB Function27/1(beta)  "beta2_C"
  MATLAB Function38/1(alpha) -> Goto73/1, MATLAB Function26/1(alpha), MATLAB Function27/2(alpha)  "alpha2_C"
  MATLAB Function39/1(cosGrid) -> Goto74/1, Matrix Multiply15/1  "cosGrid_C"
  MATLAB Function40/1(sinGrid) -> Goto72/1, Matrix Multiply16/1  "sinGric_C"
  Delay6/1 -> Sin9/1, MATLAB Function41/3(anglePllComp), Cos6/1
  MATLAB Function41/1(phaseError) -> Goto99/1  "phaseError_C"

== matlab function testing_C_functions_doubles_substituting_every_function/MATLAB Function9 ==
  data: a input; alpha output; b input; c input; beta output
function [alpha,beta] = calling_abc_to_alphabeta(a,b,c)
% coder.updateBuildInfo('addSourceFiles','abc_to_alphabeta.c');
% coder.cinclude('abc_to_alphabeta.h');
coder.updateBuildInfo('addSourceFiles','PLL_doubled.c');
coder.cinclude('PLL_doubled.h');


alpha = 0.0;
beta = 0.0;

alpha = coder.ceval('abc_to_alpha',a,b,c);
beta = coder.ceval('abc_to_beta',a,b,c);

== matlab function testing_C_functions_doubles_substituting_every_function/MATLAB Function10 ==
  data: cosGrid input; phaseError output; sinGrid input; anglePllComp input
function phaseError  = calling_phase_detector(cosGrid, sinGrid, anglePllComp)
% coder.updateBuildInfo('addSourceFiles','abc_to_alphabeta.c');
% coder.cinclude('abc_to_alphabeta.h');
coder.updateBuildInfo('addSourceFiles','PLL_doubled.c');
coder.cinclude('PLL_doubled.h');

phaseError = 0.0;

phaseError = coder.ceval('phase_detector', cosGrid, sinGrid, anglePllComp);

== matlab function testing_C_functions_doubles_substituting_every_function/MATLAB Function11 ==
  data: len input; sample input; y output; t input
function y = calling_moving_avg(len, sample, t)
% coder.updateBuildInfo('addSourceFiles','moving_avg.c');
% coder.cinclude('moving_avg.h');

coder.updateBuildInfo('addSourceFiles','MAF.c');
coder.cinclude('MAF.h');

y = 0.0;
% y = coder.ceval('moving_avg',u,t);
y = coder.ceval('maf',len, sample, t);

== matlab function testing_C_functions_doubles_substituting_every_function/MATLAB Function12 ==
  data: len input; sample input; y output; t input
function y = calling_moving_avg(len, sample, t)
% coder.updateBuildInfo('addSourceFiles','moving_avg.c');
% coder.cinclude('moving_avg.h');

coder.updateBuildInfo('addSourceFiles','MAF.c');
coder.cinclude('MAF.h');

y = 0.0;
% y = coder.ceval('moving_avg',u,t);
y = coder.ceval('maf',len, sample, t);

== matlab function testing_C_functions_doubles_substituting_every_function/MATLAB Function13 ==
  data: len input; sample input; y output; t input
function y = calling_moving_avg(len, sample, t)
% coder.updateBuildInfo('addSourceFiles','moving_avg.c');
% coder.cinclude('moving_avg.h');

coder.updateBuildInfo('addSourceFiles','MAF.c');
coder.cinclude('MAF.h');

y = 0.0;
% y = coder.ceval('moving_avg',u,t);
y = coder.ceval('maf',len, sample, t);

== matlab function testing_C_functions_doubles_substituting_every_function/MATLAB Function14 ==
  data: len input; sample input; y output; t input
function y = calling_moving_avg(len, sample, t)
% coder.updateBuildInfo('addSourceFiles','moving_avg.c');
% coder.cinclude('moving_avg.h');

coder.updateBuildInfo('addSourceFiles','MAF.c');
coder.cinclude('MAF.h');

y = 0.0;
% y = coder.ceval('moving_avg',u,t);
y = coder.ceval('maf',len, sample, t);

== matlab function testing_C_functions_doubles_substituting_every_function/MATLAB Function15 ==
  data: len input; sample input; y output; t input
function y = calling_moving_avg(len, sample, t)
% coder.updateBuildInfo('addSourceFiles','moving_avg.c');
% coder.cinclude('moving_avg.h');

coder.updateBuildInfo('addSourceFiles','MAF.c');
coder.cinclude('MAF.h');

y = 0.0;
% y = coder.ceval('moving_avg',u,t);
y = coder.ceval('maf',len, sample, t);

== matlab function testing_C_functions_doubles_substituting_every_function/MATLAB Function16 ==
  data: len input; sample input; y output; t input
function y = calling_moving_avg(len, sample, t)
% coder.updateBuildInfo('addSourceFiles','moving_avg.c');
% coder.cinclude('moving_avg.h');

coder.updateBuildInfo('addSourceFiles','MAF.c');
coder.cinclude('MAF.h');

y = 0.0;
% y = coder.ceval('moving_avg',u,t);
y = coder.ceval('maf',len, sample, t);

== matlab function testing_C_functions_doubles_substituting_every_function/MATLAB Function17 ==
  data: len input; sample input; y output; t input
function y = calling_moving_avg(len, sample, t)
% coder.updateBuildInfo('addSourceFiles','moving_avg.c');
% coder.cinclude('moving_avg.h');

coder.updateBuildInfo('addSourceFiles','MAF.c');
coder.cinclude('MAF.h');

y = 0.0;
% y = coder.ceval('moving_avg',u,t);
y = coder.ceval('maf',len, sample, t);

== matlab function testing_C_functions_doubles_substituting_every_function/MATLAB Function1 ==
  data: sample1 input; sample2 input; y1 output; t input; y2 output
function [y1, y2] = calling_moving_avg(sample1, sample2, t)
% coder.updateBuildInfo('addSourceFiles','moving_avg.c');
% coder.cinclude('moving_avg.h');

coder.updateBuildInfo('addSourceFiles','MAF_doubled.c');
coder.cinclude('MAF_doubled.h');

y1 = 0.0;
y2 = 0.0;
% y = coder.ceval('moving_avg',u,t);
% y1 = coder.ceval('maf1',len, sample1, t);
% y2 = coder.ceval('maf2',len, sample2, t);
y1 = coder.ceval('maf1', sample1, t); %explicit def of length removed
y2 = coder.ceval('maf2', sample2, t); %explicit def of length removed

== matlab function testing_C_functions_doubles_substituting_every_function/MATLAB Function18 ==
  data: sample1 input; sample2 input; y1 output; t input; y2 output
function [y1, y2] = calling_moving_avg(sample1, sample2, t)
% coder.updateBuildInfo('addSourceFiles','moving_avg.c');
% coder.cinclude('moving_avg.h');

coder.updateBuildInfo('addSourceFiles','MAF_doubled.c');
coder.cinclude('MAF_doubled.h');

y1 = 0.0;
y2 = 0.0;
% y = coder.ceval('moving_avg',u,t);
% y1 = coder.ceval('maf1',len, sample1, t);
% y2 = coder.ceval('maf2',len, sample2, t);
y1 = coder.ceval('maf1', sample1, t); %explicit def of length removed
y2 = coder.ceval('maf2', sample2, t); %explicit def of length removed

== matlab function testing_C_functions_doubles_substituting_every_function/MATLAB Function21 ==
  data: a input; b input; c input; anglePll output; feedForward input; ki input; kp input; kPhi input; t input; Ts input; angle input
function anglePll  = calling_pll(a, b, c, feedForward, ki, kp, kPhi, t, Ts, angle)
% coder.updateBuildInfo('addSourceFiles','abc_to_alphabeta.c');
% coder.cinclude('abc_to_alphabeta.h');
coder.updateBuildInfo('addSourceFiles','PLL.c');
coder.cinclude('PLL.h');

anglePll = 0.0;

anglePll = coder.ceval('pll', a, b, c, feedForward, ki, kp, kPhi, t, Ts, angle);

== matlab function testing_C_functions_doubles_substituting_every_function/MATLAB Function19 ==
  data: alpha input; cos_grid output; beta input
function cos_grid = cos_grid(alpha, beta)

cos_grid = alpha/sqrt(alpha^2+beta^2);

== matlab function testing_C_functions_doubles_substituting_every_function/MATLAB Function20 ==
  data: beta input; alpha input; sin_grid output
function sin_grid = sin_grid(beta, alpha)

sin_grid = beta/sqrt(alpha^2+beta^2);

== matlab function testing_C_functions_doubles_substituting_every_function/MATLAB Function22 ==
  data: alpha input; cos_grid output; beta input
function cos_grid = cos_grid(alpha, beta)

cos_grid = alpha/sqrt(alpha^2+beta^2);

== matlab function testing_C_functions_doubles_substituting_every_function/MATLAB Function23 ==
  data: beta input; alpha input; sin_grid output
function sin_grid = sin_grid(beta, alpha)

sin_grid = beta/sqrt(alpha^2+beta^2);

== matlab function testing_C_functions_doubles_substituting_every_function/MATLAB Function24 ==
  data: alpha input; cos_grid output; beta input
function cos_grid = cos_grid(alpha, beta)

cos_grid = alpha/sqrt(alpha^2+beta^2);

== matlab function testing_C_functions_doubles_substituting_every_function/MATLAB Function25 ==
  data: beta input; alpha input; sin_grid output
function sin_grid = sin_grid(beta, alpha)

sin_grid = beta/sqrt(alpha^2+beta^2);

== matlab function testing_C_functions_doubles_substituting_every_function/MATLAB Function26 ==
  data: alpha input; cos_grid output; beta input
function cos_grid = cos_grid(alpha, beta)

cos_grid = alpha/sqrt(alpha^2+beta^2);

== matlab function testing_C_functions_doubles_substituting_every_function/MATLAB Function27 ==
  data: beta input; alpha input; sin_grid output
function sin_grid = sin_grid(beta, alpha)

sin_grid = beta/sqrt(alpha^2+beta^2);

== matlab function testing_C_functions_doubles_substituting_every_function/MATLAB Function28 ==
  data: alpha input; cos_grid output; beta input
function cos_grid = cos_grid(alpha, beta)

cos_grid = alpha/sqrt(alpha^2+beta^2);

== matlab function testing_C_functions_doubles_substituting_every_function/MATLAB Function2 ==
  data: a input; alpha output; b input; c input; beta output
function [alpha,beta] = calling_abc_to_alphabeta(a,b,c)
% coder.updateBuildInfo('addSourceFiles','abc_to_alphabeta.c');
% coder.cinclude('abc_to_alphabeta.h');
coder.updateBuildInfo('addSourceFiles','PLL_doubled.c');
coder.cinclude('PLL_doubled.h');


alpha = 0.0;
beta = 0.0;

alpha = coder.ceval('abc_to_alpha',a,b,c);
beta = coder.ceval('abc_to_beta',a,b,c);

== matlab function testing_C_functions_doubles_substituting_every_function/MATLAB Function29 ==
  data: beta input; alpha input; sin_grid output
function sin_grid = sin_grid(beta, alpha)

sin_grid = beta/sqrt(alpha^2+beta^2);

== matlab function testing_C_functions_doubles_substituting_every_function/MATLAB Function30 ==
  data: alpha input; cos_grid output; beta input
function cos_grid = cos_grid(alpha, beta)

cos_grid = alpha/sqrt(alpha^2+beta^2);

== matlab function testing_C_functions_doubles_substituting_every_function/MATLAB Function31 ==
  data: beta input; alpha input; sin_grid output
function sin_grid = sin_grid(beta, alpha)

sin_grid = beta/sqrt(alpha^2+beta^2);

== matlab function testing_C_functions_doubles_substituting_every_function/MATLAB Function32 ==
  data: alpha input; cos_grid output; beta input
function cos_grid = cos_grid(alpha, beta)

cos_grid = alpha/sqrt(alpha^2+beta^2);

== matlab function testing_C_functions_doubles_substituting_every_function/MATLAB Function33 ==
  data: beta input; alpha input; sin_grid output
function sin_grid = sin_grid(beta, alpha)

sin_grid = beta/sqrt(alpha^2+beta^2);

== matlab function testing_C_functions_doubles_substituting_every_function/MATLAB Function34 ==
  data: alpha input; d output; beta input; angle input; q output
function [d, q] = calling_alphabeta_to_dq(alpha, beta, angle)
% coder.updateBuildInfo('addSourceFiles','abc_to_alphabeta.c');
% coder.cinclude('abc_to_alphabeta.h');
coder.updateBuildInfo('addSourceFiles','PLL_doubled.c');
coder.cinclude('PLL_doubled.h');


d = 0.0;
q = 0.0;

d = coder.ceval('alphabeta_to_d',alpha, beta, angle);
q = coder.ceval('alphabeta_to_q',alpha, beta, angle);

== matlab function testing_C_functions_doubles_substituting_every_function/MATLAB Function35 ==
  data: alpha input; cos_grid output; beta input
function cos_grid = cos_grid(alpha, beta)

cos_grid = alpha/sqrt(alpha^2+beta^2);

== matlab function testing_C_functions_doubles_substituting_every_function/MATLAB Function36 ==
  data: beta input; alpha input; sin_grid output
function sin_grid = sin_grid(beta, alpha)

sin_grid = beta/sqrt(alpha^2+beta^2);

== matlab function testing_C_functions_doubles_substituting_every_function/MATLAB Function37 ==
  data: sample1 input; sample2 input; y1 output; t input; y2 output
function [y1, y2] = calling_moving_avg(sample1, sample2, t)
% coder.updateBuildInfo('addSourceFiles','moving_avg.c');
% coder.cinclude('moving_avg.h');

coder.updateBuildInfo('addSourceFiles','MAF_doubled.c');
coder.cinclude('MAF_doubled.h');

y1 = 0.0;
y2 = 0.0;
% y = coder.ceval('moving_avg',u,t);
% y1 = coder.ceval('maf1',len, sample1, t);
% y2 = coder.ceval('maf2',len, sample2, t);
y1 = coder.ceval('maf1', sample1, t); %explicit def of length removed
y2 = coder.ceval('maf2', sample2, t); %explicit def of length removed

== matlab function testing_C_functions_doubles_substituting_every_function/MATLAB Function38 ==
  data: d input; alpha output; q input; angle input; beta output
function [alpha, beta] = calling_dq_to_alphabeta(d, q, angle)
% coder.updateBuildInfo('addSourceFiles','abc_to_alphabeta.c');
% coder.cinclude('abc_to_alphabeta.h');
coder.updateBuildInfo('addSourceFiles','PLL_doubled.c');
coder.cinclude('PLL_doubled.h');


alpha = 0.0;
beta = 0.0;

alpha = coder.ceval('dq_to_alpha', d, q, angle);
beta = coder.ceval('dq_to_beta', d, q, angle);
